simulink model "IEEE34_SPSload"  (R2021b)
settings: Solver=ode4  StartTime=0.0  StopTime=5  FixedStep=50e-6  RelTol=1e-3
PreLoadFcn:
  | pGain = 0.05; % Gain of random perturbation (pu)
  | pGainAP = 0.01; % Gain of sinusoidal active power variation (pu)
  | pGainRP = 0.01; % Gain of sinusoidal reactive power variation (pu)
  | pFreqAP = 0.03; % Frequency of sinusoidal active power variation (Hz)
  | pFreqRP = 0.03; % Frequency of sinusoidal reactive power variation (Hz)
  | 
  | init_IEEE34nodetestfeeder;
InitFcn:
  | pGain = 0.05; % Gain of random perturbation (pu)
  | pGainAP = 0.01; % Gain of sinusoidal active power variation (pu)
  | pGainRP = 0.01; % Gain of sinusoidal reactive power variation (pu)
  | pFreqAP = 0.03; % Frequency of sinusoidal active power variation (Hz)
  | pFreqRP = 0.03; % Frequency of sinusoidal reactive power variation (Hz)
  | 
  | init_IEEE34nodetestfeeder;
values from neighbouring files (symbols this model uses):
  fNom = f    (= 60)    [init_IEEE34nodetestfeeder.m]
  loadcoeff = 1.0    (= 1)    [init_IEEE34nodetestfeeder.m]
  Ts = 50e-6    (= 5e-05)    [init_IEEE34nodetestfeeder.m]
  vNomMV = VsubL    (= 24900)    [init_IEEE34nodetestfeeder.m]
  VsubL = 24.9e3    (= 24900)    [init_IEEE34nodetestfeeder.m]
  VxfmL = 4.16e3    (= 4160)    [init_IEEE34nodetestfeeder.m]
undefined symbols (not defined in the file or in its folder): Ac, Bc, Cc, Dc, find_system, j
libraries: spsSeriesRLCBranchLib x418, spsGroundLib x242, simulink_extras x176, spsVoltageMeasurementLib x106, spsRMSLib x96, spsControlledCurrentSourceLib x94, spsThreePhaseVIMeasurementLib x37, spsMutualInductanceLib x24, spsCurrentMeasurementLib x12, spsOnDelayLib x12, spsLinearTransformerLib x6, spsControlledVoltageSourceLib x6
(part 10 of 33)

== system IEEE34_SPSload/SM_IEEE34/DL_842-844/Load B ==
  Controlled Current Source : spsControlledCurrentSourceLib/Controlled Current Source  Initialize=on  Source_Type=AC  Amplitude=0  Phase=0  Frequency=0  Measurements=None
  Gain : Gain  Gain=-1
  Measurement list : Subsystem
  PQ : Ground
  Series RLC Branch : spsSeriesRLCBranchLib/Series RLC Branch  LConnTagsString=__new0  RConnTagsString=__new0  BranchType=R  Resistance=1e8  Inductance=1e-3  SetiL0=off  InitialCurrent=0  Capacitance=1e-6  Setx0=off  InitialVoltage=0  Measurements=None
  Voltage Measurement1 : spsVoltageMeasurementLib/Voltage Measurement  PhasorSimulation=off  OutputType=Complex  PSBequivalent=0
  model : Subsystem
  a : PMIOPort  Tag=PMCPort  Side=Left
  b : PMIOPort  Tag=PMCPort  Port=2  Side=Left
  m : Outport  InitialOutput=[0,0,0]  VectorParamsAs1DForOutWhenUnconnected=off
  wires:
  model/2(m) -> Measurement list/1(In1)
  PQ/1 -> model/2(PQ)
  Voltage Measurement1/1 -> model/1(v)
  model/1(i) -> Gain/1
  Measurement list/1(Out1) -> m/1
  Gain/1 -> Controlled Current Source/1
  connections:
  Voltage Measurement1/LConn1 -- Series RLC Branch/LConn1 -- a/RConn1 -- Controlled Current Source/RConn1
  Voltage Measurement1/LConn2 -- Series RLC Branch/RConn1 -- b/RConn1 -- Controlled Current Source/LConn1

== system IEEE34_SPSload/SM_IEEE34/DL_844-1/Load B ==
  Controlled Current Source : spsControlledCurrentSourceLib/Controlled Current Source  Initialize=on  Source_Type=AC  Amplitude=0  Phase=0  Frequency=0  Measurements=None
  Gain : Gain  Gain=-1
  Measurement list : Subsystem
  PQ : Ground
  Series RLC Branch : spsSeriesRLCBranchLib/Series RLC Branch  LConnTagsString=__new0  RConnTagsString=__new0  BranchType=R  Resistance=1e8  Inductance=1e-3  SetiL0=off  InitialCurrent=0  Capacitance=1e-6  Setx0=off  InitialVoltage=0  Measurements=None
  Voltage Measurement1 : spsVoltageMeasurementLib/Voltage Measurement  PhasorSimulation=off  OutputType=Complex  PSBequivalent=0
  model : Subsystem
  a : PMIOPort  Tag=PMCPort  Side=Left
  b : PMIOPort  Tag=PMCPort  Port=2  Side=Left
  m : Outport  InitialOutput=[0,0,0]  VectorParamsAs1DForOutWhenUnconnected=off
  wires:
  Gain/1 -> Controlled Current Source/1
  Measurement list/1(Out1) -> m/1
  model/1(i) -> Gain/1
  Voltage Measurement1/1 -> model/1(v)
  PQ/1 -> model/2(PQ)
  model/2(m) -> Measurement list/1(In1)
  connections:
  Controlled Current Source/LConn1 -- b/RConn1 -- Series RLC Branch/RConn1 -- Voltage Measurement1/LConn2
  Controlled Current Source/RConn1 -- a/RConn1 -- Series RLC Branch/LConn1 -- Voltage Measurement1/LConn1

== system IEEE34_SPSload/SM_IEEE34/DL_844-1/Load B1 ==
  Controlled Current Source : spsControlledCurrentSourceLib/Controlled Current Source  Initialize=on  Source_Type=AC  Amplitude=0  Phase=0  Frequency=0  Measurements=None
  Gain : Gain  Gain=-1
  Measurement list : Subsystem
  PQ : Ground
  Series RLC Branch : spsSeriesRLCBranchLib/Series RLC Branch  LConnTagsString=__new0  RConnTagsString=__new0  BranchType=R  Resistance=1e8  Inductance=1e-3  SetiL0=off  InitialCurrent=0  Capacitance=1e-6  Setx0=off  InitialVoltage=0  Measurements=None
  Voltage Measurement1 : spsVoltageMeasurementLib/Voltage Measurement  PhasorSimulation=off  OutputType=Complex  PSBequivalent=0
  model : Subsystem
  a : PMIOPort  Tag=PMCPort  Side=Left
  b : PMIOPort  Tag=PMCPort  Port=2  Side=Left
  m : Outport  InitialOutput=[0,0,0]  VectorParamsAs1DForOutWhenUnconnected=off
  wires:
  Gain/1 -> Controlled Current Source/1
  Measurement list/1(Out1) -> m/1
  model/1(i) -> Gain/1
  Voltage Measurement1/1 -> model/1(v)
  PQ/1 -> model/2(PQ)
  model/2(m) -> Measurement list/1(In1)
  connections:
  Controlled Current Source/LConn1 -- b/RConn1 -- Series RLC Branch/RConn1 -- Voltage Measurement1/LConn2
  Controlled Current Source/RConn1 -- a/RConn1 -- Series RLC Branch/LConn1 -- Voltage Measurement1/LConn1

== system IEEE34_SPSload/SM_IEEE34/DL_844-1/Load B2 ==
  Controlled Current Source : spsControlledCurrentSourceLib/Controlled Current Source  Initialize=on  Source_Type=AC  Amplitude=0  Phase=0  Frequency=0  Measurements=None
  Gain : Gain  Gain=-1
  Measurement list : Subsystem
  PQ : Ground
  Series RLC Branch : spsSeriesRLCBranchLib/Series RLC Branch  LConnTagsString=__new0  RConnTagsString=__new0  BranchType=R  Resistance=1e8  Inductance=1e-3  SetiL0=off  InitialCurrent=0  Capacitance=1e-6  Setx0=off  InitialVoltage=0  Measurements=None
  Voltage Measurement1 : spsVoltageMeasurementLib/Voltage Measurement  PhasorSimulation=off  OutputType=Complex  PSBequivalent=0
  model : Subsystem
  a : PMIOPort  Tag=PMCPort  Side=Left
  b : PMIOPort  Tag=PMCPort  Port=2  Side=Left
  m : Outport  InitialOutput=[0,0,0]  VectorParamsAs1DForOutWhenUnconnected=off
  wires:
  model/2(m) -> Measurement list/1(In1)
  PQ/1 -> model/2(PQ)
  Voltage Measurement1/1 -> model/1(v)
  model/1(i) -> Gain/1
  Measurement list/1(Out1) -> m/1
  Gain/1 -> Controlled Current Source/1
  connections:
  Voltage Measurement1/LConn1 -- Series RLC Branch/LConn1 -- a/RConn1 -- Controlled Current Source/RConn1
  Voltage Measurement1/LConn2 -- Series RLC Branch/RConn1 -- b/RConn1 -- Controlled Current Source/LConn1

== system IEEE34_SPSload/SM_IEEE34/DL_844-846/Load B ==
  Controlled Current Source : spsControlledCurrentSourceLib/Controlled Current Source  Initialize=on  Source_Type=AC  Amplitude=0  Phase=0  Frequency=0  Measurements=None
  Gain : Gain  Gain=-1
  Measurement list : Subsystem
  PQ : Ground
  Series RLC Branch : spsSeriesRLCBranchLib/Series RLC Branch  LConnTagsString=__new0  RConnTagsString=__new0  BranchType=R  Resistance=1e8  Inductance=1e-3  SetiL0=off  InitialCurrent=0  Capacitance=1e-6  Setx0=off  InitialVoltage=0  Measurements=None
  Voltage Measurement1 : spsVoltageMeasurementLib/Voltage Measurement  PhasorSimulation=off  OutputType=Complex  PSBequivalent=0
  model : Subsystem
  a : PMIOPort  Tag=PMCPort  Side=Left
  b : PMIOPort  Tag=PMCPort  Port=2  Side=Left
  m : Outport  InitialOutput=[0,0,0]  VectorParamsAs1DForOutWhenUnconnected=off
  wires:
  model/2(m) -> Measurement list/1(In1)
  PQ/1 -> model/2(PQ)
  Voltage Measurement1/1 -> model/1(v)
  model/1(i) -> Gain/1
  Measurement list/1(Out1) -> m/1
  Gain/1 -> Controlled Current Source/1
  connections:
  Voltage Measurement1/LConn1 -- Series RLC Branch/LConn1 -- a/RConn1 -- Controlled Current Source/RConn1
  Voltage Measurement1/LConn2 -- Series RLC Branch/RConn1 -- b/RConn1 -- Controlled Current Source/LConn1

== system IEEE34_SPSload/SM_IEEE34/DL_844-846/Load B1 ==
  Controlled Current Source : spsControlledCurrentSourceLib/Controlled Current Source  Initialize=on  Source_Type=AC  Amplitude=0  Phase=0  Frequency=0  Measurements=None
  Gain : Gain  Gain=-1
  Measurement list : Subsystem
  PQ : Ground
  Series RLC Branch : spsSeriesRLCBranchLib/Series RLC Branch  LConnTagsString=__new0  RConnTagsString=__new0  BranchType=R  Resistance=1e8  Inductance=1e-3  SetiL0=off  InitialCurrent=0  Capacitance=1e-6  Setx0=off  InitialVoltage=0  Measurements=None
  Voltage Measurement1 : spsVoltageMeasurementLib/Voltage Measurement  PhasorSimulation=off  OutputType=Complex  PSBequivalent=0
  model : Subsystem
  a : PMIOPort  Tag=PMCPort  Side=Left
  b : PMIOPort  Tag=PMCPort  Port=2  Side=Left
  m : Outport  InitialOutput=[0,0,0]  VectorParamsAs1DForOutWhenUnconnected=off
  wires:
  model/2(m) -> Measurement list/1(In1)
  PQ/1 -> model/2(PQ)
  Voltage Measurement1/1 -> model/1(v)
  model/1(i) -> Gain/1
  Measurement list/1(Out1) -> m/1
  Gain/1 -> Controlled Current Source/1
  connections:
  Voltage Measurement1/LConn1 -- Series RLC Branch/LConn1 -- a/RConn1 -- Controlled Current Source/RConn1
  Voltage Measurement1/LConn2 -- Series RLC Branch/RConn1 -- b/RConn1 -- Controlled Current Source/LConn1

== system IEEE34_SPSload/SM_IEEE34/DL_844-846/Load B2 ==
  Controlled Current Source : spsControlledCurrentSourceLib/Controlled Current Source  Initialize=on  Source_Type=AC  Amplitude=0  Phase=0  Frequency=0  Measurements=None
  Gain : Gain  Gain=-1
  Measurement list : Subsystem
  PQ : Ground
  Series RLC Branch : spsSeriesRLCBranchLib/Series RLC Branch  LConnTagsString=__new0  RConnTagsString=__new0  BranchType=R  Resistance=1e8  Inductance=1e-3  SetiL0=off  InitialCurrent=0  Capacitance=1e-6  Setx0=off  InitialVoltage=0  Measurements=None
  Voltage Measurement1 : spsVoltageMeasurementLib/Voltage Measurement  PhasorSimulation=off  OutputType=Complex  PSBequivalent=0
  model : Subsystem
  a : PMIOPort  Tag=PMCPort  Side=Left
  b : PMIOPort  Tag=PMCPort  Port=2  Side=Left
  m : Outport  InitialOutput=[0,0,0]  VectorParamsAs1DForOutWhenUnconnected=off
  wires:
  Gain/1 -> Controlled Current Source/1
  Measurement list/1(Out1) -> m/1
  model/1(i) -> Gain/1
  Voltage Measurement1/1 -> model/1(v)
  PQ/1 -> model/2(PQ)
  model/2(m) -> Measurement list/1(In1)
  connections:
  Controlled Current Source/LConn1 -- b/RConn1 -- Series RLC Branch/RConn1 -- Voltage Measurement1/LConn2
  Controlled Current Source/RConn1 -- a/RConn1 -- Series RLC Branch/LConn1 -- Voltage Measurement1/LConn1

== system IEEE34_SPSload/SM_IEEE34/DL_846-1/Load B ==
  Controlled Current Source : spsControlledCurrentSourceLib/Controlled Current Source  Initialize=on  Source_Type=AC  Amplitude=0  Phase=0  Frequency=0  Measurements=None
  Gain : Gain  Gain=-1
  Measurement list : Subsystem
  PQ : Ground
  Series RLC Branch : spsSeriesRLCBranchLib/Series RLC Branch  LConnTagsString=__new0  RConnTagsString=__new0  BranchType=R  Resistance=1e8  Inductance=1e-3  SetiL0=off  InitialCurrent=0  Capacitance=1e-6  Setx0=off  InitialVoltage=0  Measurements=None
  Voltage Measurement1 : spsVoltageMeasurementLib/Voltage Measurement  PhasorSimulation=off  OutputType=Complex  PSBequivalent=0
  model : Subsystem
  a : PMIOPort  Tag=PMCPort  Side=Left
  b : PMIOPort  Tag=PMCPort  Port=2  Side=Left
  m : Outport  InitialOutput=[0,0,0]  VectorParamsAs1DForOutWhenUnconnected=off
  wires:
  Gain/1 -> Controlled Current Source/1
  Measurement list/1(Out1) -> m/1
  model/1(i) -> Gain/1
  Voltage Measurement1/1 -> model/1(v)
  PQ/1 -> model/2(PQ)
  model/2(m) -> Measurement list/1(In1)
  connections:
  Controlled Current Source/LConn1 -- b/RConn1 -- Series RLC Branch/RConn1 -- Voltage Measurement1/LConn2
  Controlled Current Source/RConn1 -- a/RConn1 -- Series RLC Branch/LConn1 -- Voltage Measurement1/LConn1

== system IEEE34_SPSload/SM_IEEE34/DL_846-848/Load B ==
  Controlled Current Source : spsControlledCurrentSourceLib/Controlled Current Source  Initialize=on  Source_Type=AC  Amplitude=0  Phase=0  Frequency=0  Measurements=None
  Gain : Gain  Gain=-1
  Measurement list : Subsystem
  PQ : Ground
  Series RLC Branch : spsSeriesRLCBranchLib/Series RLC Branch  LConnTagsString=__new0  RConnTagsString=__new0  BranchType=R  Resistance=1e8  Inductance=1e-3  SetiL0=off  InitialCurrent=0  Capacitance=1e-6  Setx0=off  InitialVoltage=0  Measurements=None
  Voltage Measurement1 : spsVoltageMeasurementLib/Voltage Measurement  PhasorSimulation=off  OutputType=Complex  PSBequivalent=0
  model : Subsystem
  a : PMIOPort  Tag=PMCPort  Side=Left
  b : PMIOPort  Tag=PMCPort  Port=2  Side=Left
  m : Outport  InitialOutput=[0,0,0]  VectorParamsAs1DForOutWhenUnconnected=off
  wires:
  model/2(m) -> Measurement list/1(In1)
  PQ/1 -> model/2(PQ)
  Voltage Measurement1/1 -> model/1(v)
  model/1(i) -> Gain/1
  Measurement list/1(Out1) -> m/1
  Gain/1 -> Controlled Current Source/1
  connections:
  Voltage Measurement1/LConn1 -- Series RLC Branch/LConn1 -- a/RConn1 -- Controlled Current Source/RConn1
  Voltage Measurement1/LConn2 -- Series RLC Branch/RConn1 -- b/RConn1 -- Controlled Current Source/LConn1

== system IEEE34_SPSload/SM_IEEE34/DL_854-1/Load B ==
  Controlled Current Source : spsControlledCurrentSourceLib/Controlled Current Source  Initialize=on  Source_Type=AC  Amplitude=0  Phase=0  Frequency=0  Measurements=None
  Gain : Gain  Gain=-1
  Measurement list : Subsystem
  PQ : Ground
  Series RLC Branch : spsSeriesRLCBranchLib/Series RLC Branch  LConnTagsString=__new0  RConnTagsString=__new0  BranchType=R  Resistance=1e8  Inductance=1e-3  SetiL0=off  InitialCurrent=0  Capacitance=1e-6  Setx0=off  InitialVoltage=0  Measurements=None
  Voltage Measurement1 : spsVoltageMeasurementLib/Voltage Measurement  PhasorSimulation=off  OutputType=Complex  PSBequivalent=0
  model : Subsystem
  a : PMIOPort  Tag=PMCPort  Side=Left
  b : PMIOPort  Tag=PMCPort  Port=2  Side=Left
  m : Outport  InitialOutput=[0,0,0]  VectorParamsAs1DForOutWhenUnconnected=off
  wires:
  Gain/1 -> Controlled Current Source/1
  Measurement list/1(Out1) -> m/1
  model/1(i) -> Gain/1
  Voltage Measurement1/1 -> model/1(v)
  PQ/1 -> model/2(PQ)
  model/2(m) -> Measurement list/1(In1)
  connections:
  Controlled Current Source/LConn1 -- b/RConn1 -- Series RLC Branch/RConn1 -- Voltage Measurement1/LConn2
  Controlled Current Source/RConn1 -- a/RConn1 -- Series RLC Branch/LConn1 -- Voltage Measurement1/LConn1

== system IEEE34_SPSload/SM_IEEE34/DL_854-856/Load B ==
  Controlled Current Source : spsControlledCurrentSourceLib/Controlled Current Source  Initialize=on  Source_Type=AC  Amplitude=0  Phase=0  Frequency=0  Measurements=None
  Gain : Gain  Gain=-1
  Measurement list : Subsystem
  PQ : Ground
  Series RLC Branch : spsSeriesRLCBranchLib/Series RLC Branch  LConnTagsString=__new0  RConnTagsString=__new0  BranchType=R  Resistance=1e8  Inductance=1e-3  SetiL0=off  InitialCurrent=0  Capacitance=1e-6  Setx0=off  InitialVoltage=0  Measurements=None
  Voltage Measurement1 : spsVoltageMeasurementLib/Voltage Measurement  PhasorSimulation=off  OutputType=Complex  PSBequivalent=0
  model : Subsystem
  a : PMIOPort  Tag=PMCPort  Side=Left
  b : PMIOPort  Tag=PMCPort  Port=2  Side=Left
  m : Outport  InitialOutput=[0,0,0]  VectorParamsAs1DForOutWhenUnconnected=off
  wires:
  model/2(m) -> Measurement list/1(In1)
  PQ/1 -> model/2(PQ)
  Voltage Measurement1/1 -> model/1(v)
  model/1(i) -> Gain/1
  Measurement list/1(Out1) -> m/1
  Gain/1 -> Controlled Current Source/1
  connections:
  Voltage Measurement1/LConn1 -- Series RLC Branch/LConn1 -- a/RConn1 -- Controlled Current Source/RConn1
  Voltage Measurement1/LConn2 -- Series RLC Branch/RConn1 -- b/RConn1 -- Controlled Current Source/LConn1

== system IEEE34_SPSload/SM_IEEE34/DL_858-1/Load B ==
  Controlled Current Source : spsControlledCurrentSourceLib/Controlled Current Source  Initialize=on  Source_Type=AC  Amplitude=0  Phase=0  Frequency=0  Measurements=None
  Gain : Gain  Gain=-1
  Measurement list : Subsystem
  PQ : Ground
  Series RLC Branch : spsSeriesRLCBranchLib/Series RLC Branch  LConnTagsString=__new0  RConnTagsString=__new0  BranchType=R  Resistance=1e8  Inductance=1e-3  SetiL0=off  InitialCurrent=0  Capacitance=1e-6  Setx0=off  InitialVoltage=0  Measurements=None
  Voltage Measurement1 : spsVoltageMeasurementLib/Voltage Measurement  PhasorSimulation=off  OutputType=Complex  PSBequivalent=0
  model : Subsystem
  a : PMIOPort  Tag=PMCPort  Side=Left
  b : PMIOPort  Tag=PMCPort  Port=2  Side=Left
  m : Outport  InitialOutput=[0,0,0]  VectorParamsAs1DForOutWhenUnconnected=off
  wires:
  Gain/1 -> Controlled Current Source/1
  Measurement list/1(Out1) -> m/1
  model/1(i) -> Gain/1
  Voltage Measurement1/1 -> model/1(v)
  PQ/1 -> model/2(PQ)
  model/2(m) -> Measurement list/1(In1)
  connections:
  Controlled Current Source/LConn1 -- b/RConn1 -- Series RLC Branch/RConn1 -- Voltage Measurement1/LConn2
  Controlled Current Source/RConn1 -- a/RConn1 -- Series RLC Branch/LConn1 -- Voltage Measurement1/LConn1

== system IEEE34_SPSload/SM_IEEE34/DL_858-2/Load B ==
  Controlled Current Source : spsControlledCurrentSourceLib/Controlled Current Source  Initialize=on  Source_Type=AC  Amplitude=0  Phase=0  Frequency=0  Measurements=None
  Gain : Gain  Gain=-1
  Measurement list : Subsystem
  PQ : Ground
  Series RLC Branch : spsSeriesRLCBranchLib/Series RLC Branch  LConnTagsString=__new0  RConnTagsString=__new0  BranchType=R  Resistance=1e8  Inductance=1e-3  SetiL0=off  InitialCurrent=0  Capacitance=1e-6  Setx0=off  InitialVoltage=0  Measurements=None
  Voltage Measurement1 : spsVoltageMeasurementLib/Voltage Measurement  PhasorSimulation=off  OutputType=Complex  PSBequivalent=0
  model : Subsystem
  a : PMIOPort  Tag=PMCPort  Side=Left
  b : PMIOPort  Tag=PMCPort  Port=2  Side=Left
  m : Outport  InitialOutput=[0,0,0]  VectorParamsAs1DForOutWhenUnconnected=off
  wires:
  Gain/1 -> Controlled Current Source/1
  Measurement list/1(Out1) -> m/1
  model/1(i) -> Gain/1
  Voltage Measurement1/1 -> model/1(v)
  PQ/1 -> model/2(PQ)
  model/2(m) -> Measurement list/1(In1)
  connections:
  Controlled Current Source/LConn1 -- b/RConn1 -- Series RLC Branch/RConn1 -- Voltage Measurement1/LConn2
  Controlled Current Source/RConn1 -- a/RConn1 -- Series RLC Branch/LConn1 -- Voltage Measurement1/LConn1

== system IEEE34_SPSload/SM_IEEE34/DL_858-2/Load B1 ==
  Controlled Current Source : spsControlledCurrentSourceLib/Controlled Current Source  Initialize=on  Source_Type=AC  Amplitude=0  Phase=0  Frequency=0  Measurements=None
  Gain : Gain  Gain=-1
  Measurement list : Subsystem
  PQ : Ground
  Series RLC Branch : spsSeriesRLCBranchLib/Series RLC Branch  LConnTagsString=__new0  RConnTagsString=__new0  BranchType=R  Resistance=1e8  Inductance=1e-3  SetiL0=off  InitialCurrent=0  Capacitance=1e-6  Setx0=off  InitialVoltage=0  Measurements=None
  Voltage Measurement1 : spsVoltageMeasurementLib/Voltage Measurement  PhasorSimulation=off  OutputType=Complex  PSBequivalent=0
  model : Subsystem
  a : PMIOPort  Tag=PMCPort  Side=Left
  b : PMIOPort  Tag=PMCPort  Port=2  Side=Left
  m : Outport  InitialOutput=[0,0,0]  VectorParamsAs1DForOutWhenUnconnected=off
  wires:
  Gain/1 -> Controlled Current Source/1
  Measurement list/1(Out1) -> m/1
  model/1(i) -> Gain/1
  Voltage Measurement1/1 -> model/1(v)
  PQ/1 -> model/2(PQ)
  model/2(m) -> Measurement list/1(In1)
  connections:
  Controlled Current Source/LConn1 -- b/RConn1 -- Series RLC Branch/RConn1 -- Voltage Measurement1/LConn2
  Controlled Current Source/RConn1 -- a/RConn1 -- Series RLC Branch/LConn1 -- Voltage Measurement1/LConn1

== system IEEE34_SPSload/SM_IEEE34/DL_858-2/Load B2 ==
  Controlled Current Source : spsControlledCurrentSourceLib/Controlled Current Source  Initialize=on  Source_Type=AC  Amplitude=0  Phase=0  Frequency=0  Measurements=None
  Gain : Gain  Gain=-1
  Measurement list : Subsystem
  PQ : Ground
  Series RLC Branch : spsSeriesRLCBranchLib/Series RLC Branch  LConnTagsString=__new0  RConnTagsString=__new0  BranchType=R  Resistance=1e8  Inductance=1e-3  SetiL0=off  InitialCurrent=0  Capacitance=1e-6  Setx0=off  InitialVoltage=0  Measurements=None
  Voltage Measurement1 : spsVoltageMeasurementLib/Voltage Measurement  PhasorSimulation=off  OutputType=Complex  PSBequivalent=0
  model : Subsystem
  a : PMIOPort  Tag=PMCPort  Side=Left
  b : PMIOPort  Tag=PMCPort  Port=2  Side=Left
  m : Outport  InitialOutput=[0,0,0]  VectorParamsAs1DForOutWhenUnconnected=off
  wires:
  Gain/1 -> Controlled Current Source/1
  Measurement list/1(Out1) -> m/1
  model/1(i) -> Gain/1
  Voltage Measurement1/1 -> model/1(v)
  PQ/1 -> model/2(PQ)
  model/2(m) -> Measurement list/1(In1)
  connections:
  Controlled Current Source/LConn1 -- b/RConn1 -- Series RLC Branch/RConn1 -- Voltage Measurement1/LConn2
  Controlled Current Source/RConn1 -- a/RConn1 -- Series RLC Branch/LConn1 -- Voltage Measurement1/LConn1

== system IEEE34_SPSload/SM_IEEE34/DL_858-834/Load B ==
  Controlled Current Source : spsControlledCurrentSourceLib/Controlled Current Source  Initialize=on  Source_Type=AC  Amplitude=0  Phase=0  Frequency=0  Measurements=None
  Gain : Gain  Gain=-1
  Measurement list : Subsystem
  PQ : Ground
  Series RLC Branch : spsSeriesRLCBranchLib/Series RLC Branch  LConnTagsString=__new0  RConnTagsString=__new0  BranchType=R  Resistance=1e8  Inductance=1e-3  SetiL0=off  InitialCurrent=0  Capacitance=1e-6  Setx0=off  InitialVoltage=0  Measurements=None
  Voltage Measurement1 : spsVoltageMeasurementLib/Voltage Measurement  PhasorSimulation=off  OutputType=Complex  PSBequivalent=0
  model : Subsystem
  a : PMIOPort  Tag=PMCPort  Side=Left
  b : PMIOPort  Tag=PMCPort  Port=2  Side=Left
  m : Outport  InitialOutput=[0,0,0]  VectorParamsAs1DForOutWhenUnconnected=off
  wires:
  model/2(m) -> Measurement list/1(In1)
  PQ/1 -> model/2(PQ)
  Voltage Measurement1/1 -> model/1(v)
  model/1(i) -> Gain/1
  Measurement list/1(Out1) -> m/1
  Gain/1 -> Controlled Current Source/1
  connections:
  Voltage Measurement1/LConn1 -- Series RLC Branch/LConn1 -- a/RConn1 -- Controlled Current Source/RConn1
  Voltage Measurement1/LConn2 -- Series RLC Branch/RConn1 -- b/RConn1 -- Controlled Current Source/LConn1

== system IEEE34_SPSload/SM_IEEE34/DL_858-834/Load B1 ==
  Controlled Current Source : spsControlledCurrentSourceLib/Controlled Current Source  Initialize=on  Source_Type=AC  Amplitude=0  Phase=0  Frequency=0  Measurements=None
  Gain : Gain  Gain=-1
  Measurement list : Subsystem
  PQ : Ground
  Series RLC Branch : spsSeriesRLCBranchLib/Series RLC Branch  LConnTagsString=__new0  RConnTagsString=__new0  BranchType=R  Resistance=1e8  Inductance=1e-3  SetiL0=off  InitialCurrent=0  Capacitance=1e-6  Setx0=off  InitialVoltage=0  Measurements=None
  Voltage Measurement1 : spsVoltageMeasurementLib/Voltage Measurement  PhasorSimulation=off  OutputType=Complex  PSBequivalent=0
  model : Subsystem
  a : PMIOPort  Tag=PMCPort  Side=Left
  b : PMIOPort  Tag=PMCPort  Port=2  Side=Left
  m : Outport  InitialOutput=[0,0,0]  VectorParamsAs1DForOutWhenUnconnected=off
  wires:
  model/2(m) -> Measurement list/1(In1)
  PQ/1 -> model/2(PQ)
  Voltage Measurement1/1 -> model/1(v)
  model/1(i) -> Gain/1
  Measurement list/1(Out1) -> m/1
  Gain/1 -> Controlled Current Source/1
  connections:
  Voltage Measurement1/LConn1 -- Series RLC Branch/LConn1 -- a/RConn1 -- Controlled Current Source/RConn1
  Voltage Measurement1/LConn2 -- Series RLC Branch/RConn1 -- b/RConn1 -- Controlled Current Source/LConn1

== system IEEE34_SPSload/SM_IEEE34/DL_858-834/Load B2 ==
  Controlled Current Source : spsControlledCurrentSourceLib/Controlled Current Source  Initialize=on  Source_Type=AC  Amplitude=0  Phase=0  Frequency=0  Measurements=None
  Gain : Gain  Gain=-1
  Measurement list : Subsystem
  PQ : Ground
  Series RLC Branch : spsSeriesRLCBranchLib/Series RLC Branch  LConnTagsString=__new0  RConnTagsString=__new0  BranchType=R  Resistance=1e8  Inductance=1e-3  SetiL0=off  InitialCurrent=0  Capacitance=1e-6  Setx0=off  InitialVoltage=0  Measurements=None
  Voltage Measurement1 : spsVoltageMeasurementLib/Voltage Measurement  PhasorSimulation=off  OutputType=Complex  PSBequivalent=0
  model : Subsystem
  a : PMIOPort  Tag=PMCPort  Side=Left
  b : PMIOPort  Tag=PMCPort  Port=2  Side=Left
  m : Outport  InitialOutput=[0,0,0]  VectorParamsAs1DForOutWhenUnconnected=off
  wires:
  model/2(m) -> Measurement list/1(In1)
  PQ/1 -> model/2(PQ)
  Voltage Measurement1/1 -> model/1(v)
  model/1(i) -> Gain/1
  Measurement list/1(Out1) -> m/1
  Gain/1 -> Controlled Current Source/1
  connections:
  Voltage Measurement1/LConn1 -- Series RLC Branch/LConn1 -- a/RConn1 -- Controlled Current Source/RConn1
  Voltage Measurement1/LConn2 -- Series RLC Branch/RConn1 -- b/RConn1 -- Controlled Current Source/LConn1

== system IEEE34_SPSload/SM_IEEE34/DL_858-864/Load B ==
  Controlled Current Source : spsControlledCurrentSourceLib/Controlled Current Source  Initialize=on  Source_Type=AC  Amplitude=0  Phase=0  Frequency=0  Measurements=None
  Gain : Gain  Gain=-1
  Measurement list : Subsystem
  PQ : Ground
  Series RLC Branch : spsSeriesRLCBranchLib/Series RLC Branch  LConnTagsString=__new0  RConnTagsString=__new0  BranchType=R  Resistance=1e8  Inductance=1e-3  SetiL0=off  InitialCurrent=0  Capacitance=1e-6  Setx0=off  InitialVoltage=0  Measurements=None
  Voltage Measurement1 : spsVoltageMeasurementLib/Voltage Measurement  PhasorSimulation=off  OutputType=Complex  PSBequivalent=0
  model : Subsystem
  a : PMIOPort  Tag=PMCPort  Side=Left
  b : PMIOPort  Tag=PMCPort  Port=2  Side=Left
  m : Outport  InitialOutput=[0,0,0]  VectorParamsAs1DForOutWhenUnconnected=off
  wires:
  model/2(m) -> Measurement list/1(In1)
  PQ/1 -> model/2(PQ)
  Voltage Measurement1/1 -> model/1(v)
  model/1(i) -> Gain/1
  Measurement list/1(Out1) -> m/1
  Gain/1 -> Controlled Current Source/1
  connections:
  Voltage Measurement1/LConn1 -- Series RLC Branch/LConn1 -- a/RConn1 -- Controlled Current Source/RConn1
  Voltage Measurement1/LConn2 -- Series RLC Branch/RConn1 -- b/RConn1 -- Controlled Current Source/LConn1

== system IEEE34_SPSload/SM_IEEE34/DL_860-1/Load A ==
  Controlled Current Source : spsControlledCurrentSourceLib/Controlled Current Source  Initialize=on  Source_Type=AC  Amplitude=0  Phase=0  Frequency=0  Measurements=None
  Gain : Gain  Gain=-1
  Measurement list : Subsystem
  PQ : Ground
  Series RLC Branch : spsSeriesRLCBranchLib/Series RLC Branch  LConnTagsString=__new0  RConnTagsString=__new0  BranchType=R  Resistance=1e8  Inductance=1e-3  SetiL0=off  InitialCurrent=0  Capacitance=1e-6  Setx0=off  InitialVoltage=0  Measurements=None
  Voltage Measurement1 : spsVoltageMeasurementLib/Voltage Measurement  PhasorSimulation=off  OutputType=Complex  PSBequivalent=0
  model : Subsystem
  a : PMIOPort  Tag=PMCPort  Side=Left
  b : PMIOPort  Tag=PMCPort  Port=2  Side=Left
  m : Outport  InitialOutput=[0,0,0]  VectorParamsAs1DForOutWhenUnconnected=off
  wires:
  Gain/1 -> Controlled Current Source/1
  Measurement list/1(Out1) -> m/1
  model/1(i) -> Gain/1
  Voltage Measurement1/1 -> model/1(v)
  PQ/1 -> model/2(PQ)
  model/2(m) -> Measurement list/1(In1)
  connections:
  Controlled Current Source/LConn1 -- b/RConn1 -- Series RLC Branch/RConn1 -- Voltage Measurement1/LConn2
  Controlled Current Source/RConn1 -- a/RConn1 -- Series RLC Branch/LConn1 -- Voltage Measurement1/LConn1

== system IEEE34_SPSload/SM_IEEE34/DL_860-1/Load B ==
  Controlled Current Source : spsControlledCurrentSourceLib/Controlled Current Source  Initialize=on  Source_Type=AC  Amplitude=0  Phase=0  Frequency=0  Measurements=None
  Gain : Gain  Gain=-1
  Measurement list : Subsystem
  PQ : Ground
  Series RLC Branch : spsSeriesRLCBranchLib/Series RLC Branch  LConnTagsString=__new0  RConnTagsString=__new0  BranchType=R  Resistance=1e8  Inductance=1e-3  SetiL0=off  InitialCurrent=0  Capacitance=1e-6  Setx0=off  InitialVoltage=0  Measurements=None
  Voltage Measurement1 : spsVoltageMeasurementLib/Voltage Measurement  PhasorSimulation=off  OutputType=Complex  PSBequivalent=0
  model : Subsystem
  a : PMIOPort  Tag=PMCPort  Side=Left
  b : PMIOPort  Tag=PMCPort  Port=2  Side=Left
  m : Outport  InitialOutput=[0,0,0]  VectorParamsAs1DForOutWhenUnconnected=off
  wires:
  Gain/1 -> Controlled Current Source/1
  Measurement list/1(Out1) -> m/1
  model/1(i) -> Gain/1
  Voltage Measurement1/1 -> model/1(v)
  PQ/1 -> model/2(PQ)
  model/2(m) -> Measurement list/1(In1)
  connections:
  Controlled Current Source/LConn1 -- b/RConn1 -- Series RLC Branch/RConn1 -- Voltage Measurement1/LConn2
  Controlled Current Source/RConn1 -- a/RConn1 -- Series RLC Branch/LConn1 -- Voltage Measurement1/LConn1

== system IEEE34_SPSload/SM_IEEE34/DL_860-1/Load C ==
  Controlled Current Source : spsControlledCurrentSourceLib/Controlled Current Source  Initialize=on  Source_Type=AC  Amplitude=0  Phase=0  Frequency=0  Measurements=None
  Gain : Gain  Gain=-1
  Measurement list : Subsystem
  PQ : Ground
  Series RLC Branch : spsSeriesRLCBranchLib/Series RLC Branch  LConnTagsString=__new0  RConnTagsString=__new0  BranchType=R  Resistance=1e8  Inductance=1e-3  SetiL0=off  InitialCurrent=0  Capacitance=1e-6  Setx0=off  InitialVoltage=0  Measurements=None
  Voltage Measurement1 : spsVoltageMeasurementLib/Voltage Measurement  PhasorSimulation=off  OutputType=Complex  PSBequivalent=0
  model : Subsystem
  a : PMIOPort  Tag=PMCPort  Side=Left
  b : PMIOPort  Tag=PMCPort  Port=2  Side=Left
  m : Outport  InitialOutput=[0,0,0]  VectorParamsAs1DForOutWhenUnconnected=off
  wires:
  Gain/1 -> Controlled Current Source/1
  Measurement list/1(Out1) -> m/1
  model/1(i) -> Gain/1
  Voltage Measurement1/1 -> model/1(v)
  PQ/1 -> model/2(PQ)
  model/2(m) -> Measurement list/1(In1)
  connections:
  Controlled Current Source/LConn1 -- b/RConn1 -- Series RLC Branch/RConn1 -- Voltage Measurement1/LConn2
  Controlled Current Source/RConn1 -- a/RConn1 -- Series RLC Branch/LConn1 -- Voltage Measurement1/LConn1

== system IEEE34_SPSload/SM_IEEE34/DL_860-836/Load A ==
  Controlled Current Source : spsControlledCurrentSourceLib/Controlled Current Source  Initialize=on  Source_Type=AC  Amplitude=0  Phase=0  Frequency=0  Measurements=None
  Gain : Gain  Gain=-1
  Measurement list : Subsystem
  PQ : Ground
  Series RLC Branch : spsSeriesRLCBranchLib/Series RLC Branch  LConnTagsString=__new0  RConnTagsString=__new0  BranchType=R  Resistance=1e8  Inductance=1e-3  SetiL0=off  InitialCurrent=0  Capacitance=1e-6  Setx0=off  InitialVoltage=0  Measurements=None
  Voltage Measurement1 : spsVoltageMeasurementLib/Voltage Measurement  PhasorSimulation=off  OutputType=Complex  PSBequivalent=0
  model : Subsystem
  a : PMIOPort  Tag=PMCPort  Side=Left
  b : PMIOPort  Tag=PMCPort  Port=2  Side=Left
  m : Outport  InitialOutput=[0,0,0]  VectorParamsAs1DForOutWhenUnconnected=off
  wires:
  model/2(m) -> Measurement list/1(In1)
  PQ/1 -> model/2(PQ)
  Voltage Measurement1/1 -> model/1(v)
  model/1(i) -> Gain/1
  Measurement list/1(Out1) -> m/1
  Gain/1 -> Controlled Current Source/1
  connections:
  Voltage Measurement1/LConn1 -- Series RLC Branch/LConn1 -- a/RConn1 -- Controlled Current Source/RConn1
  Voltage Measurement1/LConn2 -- Series RLC Branch/RConn1 -- b/RConn1 -- Controlled Current Source/LConn1

== system IEEE34_SPSload/SM_IEEE34/DL_860-836/Load B ==
  Controlled Current Source : spsControlledCurrentSourceLib/Controlled Current Source  Initialize=on  Source_Type=AC  Amplitude=0  Phase=0  Frequency=0  Measurements=None
  Gain : Gain  Gain=-1
  Measurement list : Subsystem
  PQ : Ground
  Series RLC Branch : spsSeriesRLCBranchLib/Series RLC Branch  LConnTagsString=__new0  RConnTagsString=__new0  BranchType=R  Resistance=1e8  Inductance=1e-3  SetiL0=off  InitialCurrent=0  Capacitance=1e-6  Setx0=off  InitialVoltage=0  Measurements=None
  Voltage Measurement1 : spsVoltageMeasurementLib/Voltage Measurement  PhasorSimulation=off  OutputType=Complex  PSBequivalent=0
  model : Subsystem
  a : PMIOPort  Tag=PMCPort  Side=Left
  b : PMIOPort  Tag=PMCPort  Port=2  Side=Left
  m : Outport  InitialOutput=[0,0,0]  VectorParamsAs1DForOutWhenUnconnected=off
  wires:
  model/2(m) -> Measurement list/1(In1)
  PQ/1 -> model/2(PQ)
  Voltage Measurement1/1 -> model/1(v)
  model/1(i) -> Gain/1
  Measurement list/1(Out1) -> m/1
  Gain/1 -> Controlled Current Source/1
  connections:
  Voltage Measurement1/LConn1 -- Series RLC Branch/LConn1 -- a/RConn1 -- Controlled Current Source/RConn1
  Voltage Measurement1/LConn2 -- Series RLC Branch/RConn1 -- b/RConn1 -- Controlled Current Source/LConn1

== system IEEE34_SPSload/SM_IEEE34/DL_860-836/Load C ==
  Controlled Current Source : spsControlledCurrentSourceLib/Controlled Current Source  Initialize=on  Source_Type=AC  Amplitude=0  Phase=0  Frequency=0  Measurements=None
  Gain : Gain  Gain=-1
  Measurement list : Subsystem
  PQ : Ground
  Series RLC Branch : spsSeriesRLCBranchLib/Series RLC Branch  LConnTagsString=__new0  RConnTagsString=__new0  BranchType=R  Resistance=1e8  Inductance=1e-3  SetiL0=off  InitialCurrent=0  Capacitance=1e-6  Setx0=off  InitialVoltage=0  Measurements=None
  Voltage Measurement1 : spsVoltageMeasurementLib/Voltage Measurement  PhasorSimulation=off  OutputType=Complex  PSBequivalent=0
  model : Subsystem
  a : PMIOPort  Tag=PMCPort  Side=Left
  b : PMIOPort  Tag=PMCPort  Port=2  Side=Left
  m : Outport  InitialOutput=[0,0,0]  VectorParamsAs1DForOutWhenUnconnected=off
  wires:
  model/2(m) -> Measurement list/1(In1)
  PQ/1 -> model/2(PQ)
  Voltage Measurement1/1 -> model/1(v)
  model/1(i) -> Gain/1
  Measurement list/1(Out1) -> m/1
  Gain/1 -> Controlled Current Source/1
  connections:
  Voltage Measurement1/LConn1 -- Series RLC Branch/LConn1 -- a/RConn1 -- Controlled Current Source/RConn1
  Voltage Measurement1/LConn2 -- Series RLC Branch/RConn1 -- b/RConn1 -- Controlled Current Source/LConn1

== system IEEE34_SPSload/SM_IEEE34/Regulator 1/Single Phase SVR_A ==
  Line Drop Compensator : Subsystem
  Transformer with Taps : Subsystem
  Voltage Regulator Control : Subsystem
  S : PMIOPort  Tag=PMCPort  Side=Left
  L : PMIOPort  Tag=PMCPort  Port=2  Side=Right
  Tap : Outport  VectorParamsAs1DForOutWhenUnconnected=off
  tag scope: Vr1a=global
  wires:
  Transformer with Taps/2(Vsec) -> Line Drop Compensator/2(Vsec)
  Transformer with Taps/1(Isec) -> Line Drop Compensator/1(Isec)
  Voltage Regulator Control/1(N) -> Transformer with Taps/1(N)
  Voltage Regulator Control/2(Tap) -> Tap/1
  Line Drop Compensator/1(Vm) -> [Vr1a], Voltage Regulator Control/1(Vm)
  connections:
  S/RConn1 -- Transformer with Taps/LConn1
  Transformer with Taps/RConn1 -- L/RConn1

== system IEEE34_SPSload/SM_IEEE34/Regulator 1/Single Phase SVR_B ==
  Line Drop Compensator : Subsystem
  Transformer with Taps : Subsystem
  Voltage Regulator Control : Subsystem
  S : PMIOPort  Tag=PMCPort  Side=Left
  L : PMIOPort  Tag=PMCPort  Port=2  Side=Right
  Tap : Outport  VectorParamsAs1DForOutWhenUnconnected=off
  tag scope: Vr1b=global
  wires:
  Line Drop Compensator/1(Vm) -> Voltage Regulator Control/1(Vm), [Vr1b]
  Voltage Regulator Control/2(Tap) -> Tap/1
  Voltage Regulator Control/1(N) -> Transformer with Taps/1(N)
  Transformer with Taps/1(Isec) -> Line Drop Compensator/1(Isec)
  Transformer with Taps/2(Vsec) -> Line Drop Compensator/2(Vsec)
  connections:
  Transformer with Taps/RConn1 -- L/RConn1
  S/RConn1 -- Transformer with Taps/LConn1

== system IEEE34_SPSload/SM_IEEE34/Regulator 1/Single Phase SVR_C ==
  Line Drop Compensator : Subsystem
  Transformer with Taps : Subsystem
  Voltage Regulator Control : Subsystem
  S : PMIOPort  Tag=PMCPort  Side=Left
  L : PMIOPort  Tag=PMCPort  Port=2  Side=Right
  Tap : Outport  VectorParamsAs1DForOutWhenUnconnected=off
  tag scope: Vr1c=global
  wires:
  Transformer with Taps/2(Vsec) -> Line Drop Compensator/2(Vsec)
  Transformer with Taps/1(Isec) -> Line Drop Compensator/1(Isec)
  Voltage Regulator Control/1(N) -> Transformer with Taps/1(N)
  Voltage Regulator Control/2(Tap) -> Tap/1
  Line Drop Compensator/1(Vm) -> [Vr1c], Voltage Regulator Control/1(Vm)
  connections:
  S/RConn1 -- Transformer with Taps/LConn1
  Transformer with Taps/RConn1 -- L/RConn1

== system IEEE34_SPSload/SM_IEEE34/Regulator 2/Single Phase SVR_A ==
  Line Drop Compensator : Subsystem
  Transformer with Taps : Subsystem
  Voltage Regulator Control : Subsystem
  S : PMIOPort  Tag=PMCPort  Side=Left
  L : PMIOPort  Tag=PMCPort  Port=2  Side=Right
  Tap : Outport  VectorParamsAs1DForOutWhenUnconnected=off
  tag scope: Vr2a=global
  wires:
  Transformer with Taps/2(Vsec) -> Line Drop Compensator/2(Vsec)
  Transformer with Taps/1(Isec) -> Line Drop Compensator/1(Isec)
  Voltage Regulator Control/1(N) -> Transformer with Taps/1(N)
  Voltage Regulator Control/2(Tap) -> Tap/1
  Line Drop Compensator/1(Vm) -> Voltage Regulator Control/1(Vm), [Vr2a]
  connections:
  S/RConn1 -- Transformer with Taps/LConn1
  Transformer with Taps/RConn1 -- L/RConn1

== system IEEE34_SPSload/SM_IEEE34/Regulator 2/Single Phase SVR_B ==
  Line Drop Compensator : Subsystem
  Transformer with Taps : Subsystem
  Voltage Regulator Control : Subsystem
  S : PMIOPort  Tag=PMCPort  Side=Left
  L : PMIOPort  Tag=PMCPort  Port=2  Side=Right
  Tap : Outport  VectorParamsAs1DForOutWhenUnconnected=off
  tag scope: Vr2b=global
  wires:
  Line Drop Compensator/1(Vm) -> [Vr2b], Voltage Regulator Control/1(Vm)
  Voltage Regulator Control/2(Tap) -> Tap/1
  Voltage Regulator Control/1(N) -> Transformer with Taps/1(N)
  Transformer with Taps/1(Isec) -> Line Drop Compensator/1(Isec)
  Transformer with Taps/2(Vsec) -> Line Drop Compensator/2(Vsec)
  connections:
  Transformer with Taps/RConn1 -- L/RConn1
  S/RConn1 -- Transformer with Taps/LConn1

== system IEEE34_SPSload/SM_IEEE34/Regulator 2/Single Phase SVR_C ==
  Line Drop Compensator : Subsystem
  Transformer with Taps : Subsystem
  Voltage Regulator Control : Subsystem
  S : PMIOPort  Tag=PMCPort  Side=Left
  L : PMIOPort  Tag=PMCPort  Port=2  Side=Right
  Tap : Outport  VectorParamsAs1DForOutWhenUnconnected=off
  tag scope: Vr2c=global
  wires:
  Transformer with Taps/2(Vsec) -> Line Drop Compensator/2(Vsec)
  Transformer with Taps/1(Isec) -> Line Drop Compensator/1(Isec)
  Voltage Regulator Control/1(N) -> Transformer with Taps/1(N)
  Voltage Regulator Control/2(Tap) -> Tap/1
  Line Drop Compensator/1(Vm) -> Voltage Regulator Control/1(Vm), [Vr2c]
  connections:
  S/RConn1 -- Transformer with Taps/LConn1
  Transformer with Taps/RConn1 -- L/RConn1

== system IEEE34_SPSload/SM_IEEE34/Spot 830/Load B ==
  Controlled Current Source : spsControlledCurrentSourceLib/Controlled Current Source  Initialize=on  Source_Type=AC  Amplitude=0  Phase=0  Frequency=0  Measurements=None
  Gain : Gain  Gain=-1
  Measurement list : Subsystem
  PQ : Ground
  Series RLC Branch : spsSeriesRLCBranchLib/Series RLC Branch  LConnTagsString=__new0  RConnTagsString=__new0  BranchType=R  Resistance=1e8  Inductance=1e-3  SetiL0=off  InitialCurrent=0  Capacitance=1e-6  Setx0=off  InitialVoltage=0  Measurements=None
  Voltage Measurement1 : spsVoltageMeasurementLib/Voltage Measurement  PhasorSimulation=off  OutputType=Complex  PSBequivalent=0
  model : Subsystem
  a : PMIOPort  Tag=PMCPort  Side=Left
  b : PMIOPort  Tag=PMCPort  Port=2  Side=Left
  m : Outport  InitialOutput=[0,0,0]  VectorParamsAs1DForOutWhenUnconnected=off
  wires:
  model/2(m) -> Measurement list/1(In1)
  PQ/1 -> model/2(PQ)
  Voltage Measurement1/1 -> model/1(v)
  model/1(i) -> Gain/1
  Measurement list/1(Out1) -> m/1
  Gain/1 -> Controlled Current Source/1
  connections:
  Voltage Measurement1/LConn1 -- Series RLC Branch/LConn1 -- a/RConn1 -- Controlled Current Source/RConn1
  Voltage Measurement1/LConn2 -- Series RLC Branch/RConn1 -- b/RConn1 -- Controlled Current Source/LConn1

== system IEEE34_SPSload/SM_IEEE34/Spot 830/Load B1 ==
  Controlled Current Source : spsControlledCurrentSourceLib/Controlled Current Source  Initialize=on  Source_Type=AC  Amplitude=0  Phase=0  Frequency=0  Measurements=None
  Gain : Gain  Gain=-1
  Measurement list : Subsystem
  PQ : Ground
  Series RLC Branch : spsSeriesRLCBranchLib/Series RLC Branch  LConnTagsString=__new0  RConnTagsString=__new0  BranchType=R  Resistance=1e8  Inductance=1e-3  SetiL0=off  InitialCurrent=0  Capacitance=1e-6  Setx0=off  InitialVoltage=0  Measurements=None
  Voltage Measurement1 : spsVoltageMeasurementLib/Voltage Measurement  PhasorSimulation=off  OutputType=Complex  PSBequivalent=0
  model : Subsystem
  a : PMIOPort  Tag=PMCPort  Side=Left
  b : PMIOPort  Tag=PMCPort  Port=2  Side=Left
  m : Outport  InitialOutput=[0,0,0]  VectorParamsAs1DForOutWhenUnconnected=off
  wires:
  model/2(m) -> Measurement list/1(In1)
  PQ/1 -> model/2(PQ)
  Voltage Measurement1/1 -> model/1(v)
  model/1(i) -> Gain/1
  Measurement list/1(Out1) -> m/1
  Gain/1 -> Controlled Current Source/1
  connections:
  Voltage Measurement1/LConn1 -- Series RLC Branch/LConn1 -- a/RConn1 -- Controlled Current Source/RConn1
  Voltage Measurement1/LConn2 -- Series RLC Branch/RConn1 -- b/RConn1 -- Controlled Current Source/LConn1

== system IEEE34_SPSload/SM_IEEE34/Spot 830/Load B2 ==
  Controlled Current Source : spsControlledCurrentSourceLib/Controlled Current Source  Initialize=on  Source_Type=AC  Amplitude=0  Phase=0  Frequency=0  Measurements=None
  Gain : Gain  Gain=-1
  Measurement list : Subsystem
  PQ : Ground
  Series RLC Branch : spsSeriesRLCBranchLib/Series RLC Branch  LConnTagsString=__new0  RConnTagsString=__new0  BranchType=R  Resistance=1e8  Inductance=1e-3  SetiL0=off  InitialCurrent=0  Capacitance=1e-6  Setx0=off  InitialVoltage=0  Measurements=None
  Voltage Measurement1 : spsVoltageMeasurementLib/Voltage Measurement  PhasorSimulation=off  OutputType=Complex  PSBequivalent=0
  model : Subsystem
  a : PMIOPort  Tag=PMCPort  Side=Left
  b : PMIOPort  Tag=PMCPort  Port=2  Side=Left
  m : Outport  InitialOutput=[0,0,0]  VectorParamsAs1DForOutWhenUnconnected=off
  wires:
  model/2(m) -> Measurement list/1(In1)
  PQ/1 -> model/2(PQ)
  Voltage Measurement1/1 -> model/1(v)
  model/1(i) -> Gain/1
  Measurement list/1(Out1) -> m/1
  Gain/1 -> Controlled Current Source/1
  connections:
  Voltage Measurement1/LConn1 -- Series RLC Branch/LConn1 -- a/RConn1 -- Controlled Current Source/RConn1
  Voltage Measurement1/LConn2 -- Series RLC Branch/RConn1 -- b/RConn1 -- Controlled Current Source/LConn1

== system IEEE34_SPSload/SM_IEEE34/Spot 840/Load B ==
  Controlled Current Source : spsControlledCurrentSourceLib/Controlled Current Source  Initialize=on  Source_Type=AC  Amplitude=0  Phase=0  Frequency=0  Measurements=None
  Gain : Gain  Gain=-1
  Measurement list : Subsystem
  PQ : Ground
  Series RLC Branch : spsSeriesRLCBranchLib/Series RLC Branch  LConnTagsString=__new0  RConnTagsString=__new0  BranchType=R  Resistance=1e8  Inductance=1e-3  SetiL0=off  InitialCurrent=0  Capacitance=1e-6  Setx0=off  InitialVoltage=0  Measurements=None
  Voltage Measurement1 : spsVoltageMeasurementLib/Voltage Measurement  PhasorSimulation=off  OutputType=Complex  PSBequivalent=0
  model : Subsystem
  a : PMIOPort  Tag=PMCPort  Side=Left
  b : PMIOPort  Tag=PMCPort  Port=2  Side=Left
  m : Outport  InitialOutput=[0,0,0]  VectorParamsAs1DForOutWhenUnconnected=off
  wires:
  model/2(m) -> Measurement list/1(In1)
  PQ/1 -> model/2(PQ)
  Voltage Measurement1/1 -> model/1(v)
  model/1(i) -> Gain/1
  Measurement list/1(Out1) -> m/1
  Gain/1 -> Controlled Current Source/1
  connections:
  Voltage Measurement1/LConn1 -- Series RLC Branch/LConn1 -- a/RConn1 -- Controlled Current Source/RConn1
  Voltage Measurement1/LConn2 -- Series RLC Branch/RConn1 -- b/RConn1 -- Controlled Current Source/LConn1

== system IEEE34_SPSload/SM_IEEE34/Spot 840/Load B1 ==
  Controlled Current Source : spsControlledCurrentSourceLib/Controlled Current Source  Initialize=on  Source_Type=AC  Amplitude=0  Phase=0  Frequency=0  Measurements=None
  Gain : Gain  Gain=-1
  Measurement list : Subsystem
  PQ : Ground
  Series RLC Branch : spsSeriesRLCBranchLib/Series RLC Branch  LConnTagsString=__new0  RConnTagsString=__new0  BranchType=R  Resistance=1e8  Inductance=1e-3  SetiL0=off  InitialCurrent=0  Capacitance=1e-6  Setx0=off  InitialVoltage=0  Measurements=None
  Voltage Measurement1 : spsVoltageMeasurementLib/Voltage Measurement  PhasorSimulation=off  OutputType=Complex  PSBequivalent=0
  model : Subsystem
  a : PMIOPort  Tag=PMCPort  Side=Left
  b : PMIOPort  Tag=PMCPort  Port=2  Side=Left
  m : Outport  InitialOutput=[0,0,0]  VectorParamsAs1DForOutWhenUnconnected=off
  wires:
  Gain/1 -> Controlled Current Source/1
  Measurement list/1(Out1) -> m/1
  model/1(i) -> Gain/1
  Voltage Measurement1/1 -> model/1(v)
  PQ/1 -> model/2(PQ)
  model/2(m) -> Measurement list/1(In1)
  connections:
  Controlled Current Source/LConn1 -- b/RConn1 -- Series RLC Branch/RConn1 -- Voltage Measurement1/LConn2
  Controlled Current Source/RConn1 -- a/RConn1 -- Series RLC Branch/LConn1 -- Voltage Measurement1/LConn1

== system IEEE34_SPSload/SM_IEEE34/Spot 840/Load B2 ==
  Controlled Current Source : spsControlledCurrentSourceLib/Controlled Current Source  Initialize=on  Source_Type=AC  Amplitude=0  Phase=0  Frequency=0  Measurements=None
  Gain : Gain  Gain=-1
  Measurement list : Subsystem
  PQ : Ground
  Series RLC Branch : spsSeriesRLCBranchLib/Series RLC Branch  LConnTagsString=__new0  RConnTagsString=__new0  BranchType=R  Resistance=1e8  Inductance=1e-3  SetiL0=off  InitialCurrent=0  Capacitance=1e-6  Setx0=off  InitialVoltage=0  Measurements=None
  Voltage Measurement1 : spsVoltageMeasurementLib/Voltage Measurement  PhasorSimulation=off  OutputType=Complex  PSBequivalent=0
  model : Subsystem
  a : PMIOPort  Tag=PMCPort  Side=Left
  b : PMIOPort  Tag=PMCPort  Port=2  Side=Left
  m : Outport  InitialOutput=[0,0,0]  VectorParamsAs1DForOutWhenUnconnected=off
  wires:
  model/2(m) -> Measurement list/1(In1)
  PQ/1 -> model/2(PQ)
  Voltage Measurement1/1 -> model/1(v)
  model/1(i) -> Gain/1
  Measurement list/1(Out1) -> m/1
  Gain/1 -> Controlled Current Source/1
  connections:
  Voltage Measurement1/LConn1 -- Series RLC Branch/LConn1 -- a/RConn1 -- Controlled Current Source/RConn1
  Voltage Measurement1/LConn2 -- Series RLC Branch/RConn1 -- b/RConn1 -- Controlled Current Source/LConn1

== system IEEE34_SPSload/SM_IEEE34/Spot 844/B1 ==
  Ground : spsGroundLib/Ground  LConnTagsString=a
  I : spsCurrentMeasurementLib/Current Measurement  PhasorSimulation=off  OutputType=Complex  PSBequivalent=0
  V : spsVoltageMeasurementLib/Voltage Measurement  PhasorSimulation=off  OutputType=Complex  PSBequivalent=0
  A : PMIOPort  Side=Left
  B : PMIOPort  Port=2  Side=Right
  v : Outport
  i : Outport  Port=2
  wires:
  I/1 -> i/1
  V/1 -> v/1
  connections:
  B/RConn1 -- I/RConn1
  Ground/LConn1 -- V/LConn2
  A/RConn1 -- I/LConn1 -- V/LConn1

== system IEEE34_SPSload/SM_IEEE34/Spot 844/B2 ==
  Ground : spsGroundLib/Ground  LConnTagsString=a
  I : spsCurrentMeasurementLib/Current Measurement  PhasorSimulation=off  OutputType=Complex  PSBequivalent=0
  V : spsVoltageMeasurementLib/Voltage Measurement  PhasorSimulation=off  OutputType=Complex  PSBequivalent=0
  A : PMIOPort  Side=Left
  B : PMIOPort  Port=2  Side=Right
  v : Outport
  i : Outport  Port=2
  wires:
  V/1 -> v/1
  I/1 -> i/1
  connections:
  V/LConn1 -- I/LConn1 -- A/RConn1
  Ground/LConn1 -- V/LConn2
  B/RConn1 -- I/RConn1

== system IEEE34_SPSload/SM_IEEE34/Spot 844/B864 ==
  Ground : spsGroundLib/Ground  LConnTagsString=a
  I : spsCurrentMeasurementLib/Current Measurement  PhasorSimulation=off  OutputType=Complex  PSBequivalent=0
  V : spsVoltageMeasurementLib/Voltage Measurement  PhasorSimulation=off  OutputType=Complex  PSBequivalent=0
  A : PMIOPort  Side=Left
  B : PMIOPort  Port=2  Side=Right
  v : Outport
  i : Outport  Port=2
  wires:
  V/1 -> v/1
  I/1 -> i/1
  connections:
  V/LConn1 -- I/LConn1 -- A/RConn1
  Ground/LConn1 -- V/LConn2
  B/RConn1 -- I/RConn1

== system IEEE34_SPSload/SM_IEEE34/Spot 844/Load B ==
  Controlled Current Source : spsControlledCurrentSourceLib/Controlled Current Source  Initialize=on  Source_Type=AC  Amplitude=0  Phase=0  Frequency=0  Measurements=None
  Gain : Gain  Gain=-1
  Measurement list : Subsystem
  PQ : Ground
  Series RLC Branch : spsSeriesRLCBranchLib/Series RLC Branch  LConnTagsString=__new0  RConnTagsString=__new0  BranchType=R  Resistance=1e8  Inductance=1e-3  SetiL0=off  InitialCurrent=0  Capacitance=1e-6  Setx0=off  InitialVoltage=0  Measurements=None
  Voltage Measurement1 : spsVoltageMeasurementLib/Voltage Measurement  PhasorSimulation=off  OutputType=Complex  PSBequivalent=0
  model : Subsystem
  a : PMIOPort  Tag=PMCPort  Side=Left
  b : PMIOPort  Tag=PMCPort  Port=2  Side=Left
  m : Outport  InitialOutput=[0,0,0]  VectorParamsAs1DForOutWhenUnconnected=off
  wires:
  model/2(m) -> Measurement list/1(In1)
  PQ/1 -> model/2(PQ)
  Voltage Measurement1/1 -> model/1(v)
  model/1(i) -> Gain/1
  Measurement list/1(Out1) -> m/1
  Gain/1 -> Controlled Current Source/1
  connections:
  Voltage Measurement1/LConn1 -- Series RLC Branch/LConn1 -- a/RConn1 -- Controlled Current Source/RConn1
  Voltage Measurement1/LConn2 -- Series RLC Branch/RConn1 -- b/RConn1 -- Controlled Current Source/LConn1
